simulink model "transformation_example_2"  (R2015a)
settings: Solver=ode45  StartTime=0.0  StopTime=.02  MaxStep=.00333  RelTol=1e-4
InitFcn:
  | close all;
  | clear all;
  | phase=pi/2;
StopFcn:
  | close all;
  | set(0,'defaultfigureposition',[0 0 450 450]')
  | 
  | figure(1);
  | compass(Fs);
  | axis equal;
  | title('SPACE VECTOR in stationary frame');
  | 
  | set(0,'defaultfigureposition',[750 0 450 450]')
  | figure(2)
  | compass(Fk,'r')
  | axis equal;
  | title('SPACE VECTOR in rotating frame')
undefined symbols (not defined in the file): j
libraries: simulink x1
settings Model: ExtModeTrigMode=oneshot  ExtModeArmWhenConnect=off  Creator=Dr. Syed Abdul rahman Kashif  LastModifiedBy=Dr Kashif
settings DataIOCC: LimitDataPoints=off  SignalLoggingSaveFormat=ModelDataLogs  TimeSaveName=t  OutputSaveName=Fs,Fk  SignalLoggingName=sigsOut
settings OptimizationCC: BooleanDataType=off  ExpressionDepthLimit=2147483647
settings DebuggingCC: SaveWithParameterizedLinksMsg=none  UnderspecifiedInitializationDetection=Classic  MergeDetectMultiDrivingBlocksExec=none  SignalResolutionControl=TryResolveAllWithWarning  MultiTaskDSMMsg=warning  MultiTaskCondExecSysMsg=none  FcnCallInpInsideContextMsg=UseLocalSettings  StateNameClashWarn=warning
settings HardwareCC: TargetUnknown=on
settings GRTTargetCC: CombineOutputUpdateFcns=off  GRTInterface=on

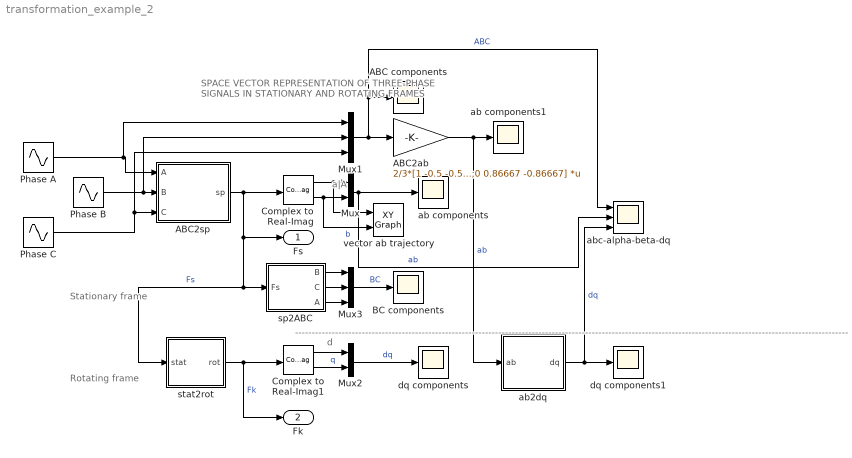
== system transformation_example_2 ==
  note: SPACE VECTOR REPRESENTATION
      | OF THREE-PHASE SIGNALS
      | IN STATIONARY AND ROTATING FRAMES
  note: a|A
  note: d
  note: Stationary frame
  note: ----------------------------------------------------------------------------------------------------------------------------------------------------------------------
  note: Rotating frame
  ABC components : Scope
      settings: TimeRange=0.02  YMin=-1  YMax=1  SampleInput=on  SampleTime=10e-6
  ABC2ab : Gain  Gain=2/3*[1 -0.5 -0.5;0 0.86667 -0.86667]  Multiplication=Matrix(K*u)  SaturateOnIntegerOverflow=on  OutDataTypeStr=Inherit: Same as input  ParamDataTypeStr=Inherit: Same as input
  ABC2sp : Subsystem
  BC components : Scope
      settings: TimeRange=0.02  YMin=-1  YMax=1
  Complex to Real-Imag : ComplexToRealImag
  Complex to Real-Imag1 : ComplexToRealImag
  Mux : Mux  Inputs=2
  Mux1 : Mux  Inputs=3
  Mux2 : Mux  Inputs=2
  Mux3 : Mux  Inputs=3
  "Phase A " : Sin  Frequency=2*pi*50  Phase=phase  SampleTime=0
  Phase B : Sin  Frequency=2*pi*50  Phase=2*pi/3+phase  SampleTime=0
  Phase C : Sin  Frequency=2*pi*50  Phase=4*pi/3+phase  SampleTime=0
  ab components : Scope
      settings: TimeRange=0.02  YMin=-1  YMax=1
  ab components1 : Scope
      settings: TimeRange=0.02  YMin=-0.5  YMax=1.5
  ab2dq : Subsystem
  abc-alpha-beta-dq : Scope  NumInputPorts=3
      settings: TimeRange=0.02  YMin=-1.25~-1.25~-0.5  YMax=1.25~1.25~1.25  SampleInput=on
  dq components : Scope
      settings: TimeRange=0.02  YMin=-1  YMax=1
  dq components1 : Scope
      settings: TimeRange=0.02  YMin=-0.2  YMax=1.2
  sp2ABC : Subsystem
  stat2rot : Subsystem
  vector ab trajectory : simulink/Sinks/XY Graph  xmin=-1  xmax=1  ymin=-1  ymax=1  st=-1
  Fs : Outport
  Fk : Outport  Port=2
  wires:
  Mux/1 -> abc-alpha-beta-dq/2, ab components/1  "ab"
  Complex to Real-Imag/1 -> Mux/1, vector ab trajectory/1
  Complex to Real-Imag/2 -> Mux/2, vector ab trajectory/2  "b"
  Mux1/1 -> ABC2ab/1, abc-alpha-beta-dq/1, ABC components/1  "ABC"
  Mux2/1 -> dq components/1  "dq"
  Complex to Real-Imag1/2 -> Mux2/2  "q"
  Complex to Real-Imag1/1 -> Mux2/1
  ABC2ab/1 -> ab components1/1, ab2dq/1(ab)  "ab"
  ab2dq/1(dq) -> abc-alpha-beta-dq/3, dq components1/1  "dq"
  sp2ABC/1(B) -> Mux3/1
  sp2ABC/2(C) -> Mux3/2
  Mux3/1 -> BC components/1  "BC"
  ABC2sp/1(sp) -> Complex to Real-Imag/1, Fs/1, sp2ABC/1(Fs), stat2rot/1(stat)  "Fs"
  stat2rot/1(rot) -> Complex to Real-Imag1/1, Fk/1  "Fk"
  sp2ABC/3(A) -> Mux3/3
  Phase C/1 -> Mux1/3, ABC2sp/3(C)
  Phase B/1 -> Mux1/2, ABC2sp/2(B)
  "Phase A "/1 -> Mux1/1, ABC2sp/1(A)

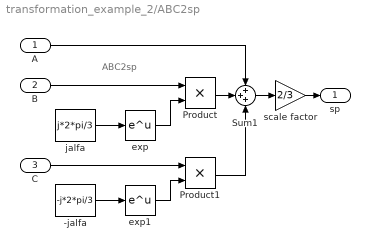
== system transformation_example_2/ABC2sp ==
  note: ABC2sp
  A : Inport
  B : Inport  Port=2
  C : Inport  Port=3
  -jalfa : Constant  Value=-j*2*pi/3
  Product : Product  SaturateOnIntegerOverflow=on  InputSameDT=on  OutDataTypeStr=Inherit: Same as first input
  Product1 : Product  SaturateOnIntegerOverflow=on  InputSameDT=on  OutDataTypeStr=Inherit: Same as first input
  Sum1 : Sum  Inputs=+++  SaturateOnIntegerOverflow=on  InputSameDT=on  OutDataTypeStr=Inherit: Same as first input
  exp : Math  SaturateOnIntegerOverflow=on
  exp1 : Math  SaturateOnIntegerOverflow=on
  jalfa : Constant  Value=j*2*pi/3
  scale factor : Gain  Gain=2/3  SaturateOnIntegerOverflow=on  OutDataTypeStr=Inherit: Same as input  ParamDataTypeStr=Inherit: Same as input
  sp : Outport
  wires:
  exp/1 -> Product/2
  jalfa/1 -> exp/1
  Product/1 -> Sum1/2
  exp1/1 -> Product1/2
  -jalfa/1 -> exp1/1
  Product1/1 -> Sum1/3
  B/1 -> Product/1
  C/1 -> Product1/1
  Sum1/1 -> scale factor/1
  scale factor/1 -> sp/1
  A/1 -> Sum1/1

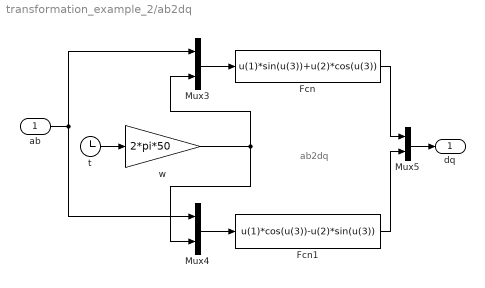
== system transformation_example_2/ab2dq ==
  note: ab2dq
  ab : Inport
  Fcn : Fcn  Expr=u(1)*sin(u(3))+u(2)*cos(u(3))
  Fcn1 : Fcn  Expr=u(1)*cos(u(3))-u(2)*sin(u(3))
  Mux3 : Mux  Inputs=2
  Mux4 : Mux  Inputs=2
  Mux5 : Mux  Inputs=2
  t : Clock
  w : Gain  Gain=2*pi*50  SaturateOnIntegerOverflow=on  OutDataTypeStr=Inherit: Same as input  ParamDataTypeStr=Inherit: Same as input
  dq : Outport
  wires:
  t/1 -> w/1
  Mux3/1 -> Fcn/1
  Mux4/1 -> Fcn1/1
  w/1 -> Mux4/2, Mux3/2
  ab/1 -> Mux4/1, Mux3/1
  Fcn1/1 -> Mux5/2
  Fcn/1 -> Mux5/1
  Mux5/1 -> dq/1

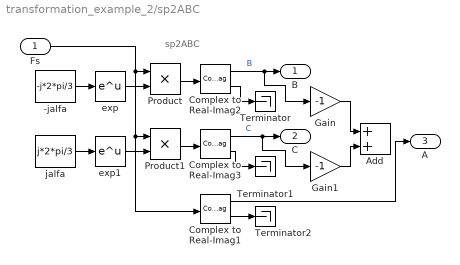
== system transformation_example_2/sp2ABC ==
  note: sp2ABC
  Fs : Inport
  -jalfa : Constant  Value=-j*2*pi/3
  Add : Sum
  Complex to Real-Imag1 : ComplexToRealImag
  Complex to Real-Imag2 : ComplexToRealImag
  Complex to Real-Imag3 : ComplexToRealImag
  Gain : Gain  Gain=-1
  Gain1 : Gain  Gain=-1
  Product : Product  SaturateOnIntegerOverflow=on  InputSameDT=on  OutDataTypeStr=Inherit: Same as first input
  Product1 : Product  SaturateOnIntegerOverflow=on  InputSameDT=on  OutDataTypeStr=Inherit: Same as first input
  Terminator : Terminator
  Terminator1 : Terminator
  Terminator2 : Terminator
  exp : Math  SaturateOnIntegerOverflow=on
  exp1 : Math  SaturateOnIntegerOverflow=on
  jalfa : Constant  Value=j*2*pi/3
  B : Outport
  C : Outport  Port=2
  A : Outport  Port=3
  wires:
  exp/1 -> Product/2
  Product/1 -> Complex to Real-Imag2/1
  Complex to Real-Imag2/2 -> Terminator/1
  -jalfa/1 -> exp/1
  Complex to Real-Imag2/1 -> Gain/1, B/1  "B"
  Fs/1 -> Product/1, Complex to Real-Imag1/1, Product1/1
  exp1/1 -> Product1/2
  Product1/1 -> Complex to Real-Imag3/1
  Complex to Real-Imag3/2 -> Terminator1/1
  jalfa/1 -> exp1/1
  Complex to Real-Imag3/1 -> Gain1/1, C/1  "C"
  Gain/1 -> Add/1
  Gain1/1 -> Add/2
  Complex to Real-Imag1/1 -> A/1
  Complex to Real-Imag1/2 -> Terminator2/1

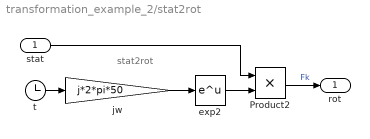
== system transformation_example_2/stat2rot ==
  note: stat2rot
  stat : Inport
  Product2 : Product  SaturateOnIntegerOverflow=on  InputSameDT=on  OutDataTypeStr=Inherit: Same as first input
  exp2 : Math  SaturateOnIntegerOverflow=on
  jw : Gain  Gain=j*2*pi*50  SaturateOnIntegerOverflow=on  OutDataTypeStr=Inherit: Same as input  ParamDataTypeStr=Inherit: Same as input
  t : Clock
  rot : Outport
  wires:
  exp2/1 -> Product2/2
  jw/1 -> exp2/1
  t/1 -> jw/1
  Product2/1 -> rot/1  "Fk"
  stat/1 -> Product2/1
